simulink model "hw3_a_LMS_model_c0"  (R2024b)
settings: Solver=ode4  StartTime=0.0  StopTime=sim_time  FixedStep=sample_time  RelTol=1e-3
values from neighbouring files (symbols this model uses):
  a = -0.8    [hw3_a_rls_v2.m]    (also in hw3_b_rls_v2.m)
  b = 0.5    [hw3_a_rls_v2.m]    (also in hw3_b_rls_v2.m)
  c = -0.5    [hw3_a_rls_v2.m]    (also in hw3_b_rls_v2.m = 0)
  noise_mean = 0    [hw3_a_rls_v2.m]    (also in hw3_b_rls_v2.m)
  noise_seed = round(rand*1e5)    [hw3_a_rls_v2.m]    (also in hw3_b_rls_v2.m)
  noise_variance = 0.5    [hw3_a_rls_v2.m]    (also in hw3_b_rls_v2.m)
  sample_time = 1    [hw3_a_rls_v2.m]    (also in hw3_b_rls_v2.m)
  Theta_0 = [0;0;0]    [hw3_a_rls_v2.m]    (also in hw3_b_rls_v2.m)
settings Model: Creator=kemal  LastModifiedBy=kemal

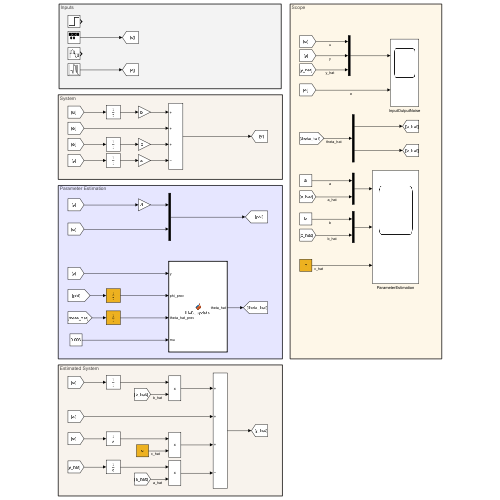
[thumbnail: Simulink's stored preview of the top-level diagram]
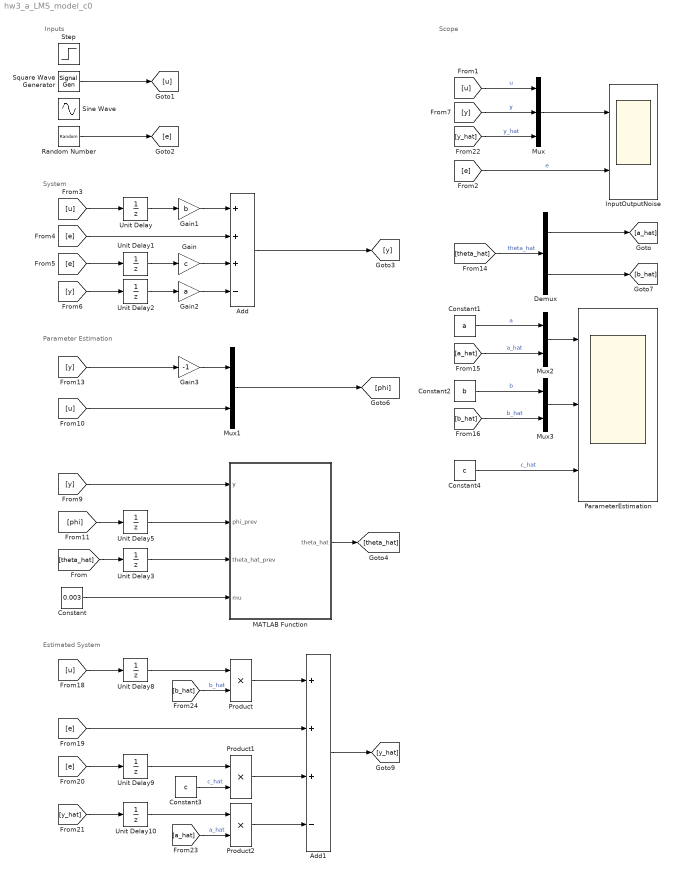
== system hw3_a_LMS_model_c0 ==
  note: Inputs
  note: System
  note: Scope
  note: Parameter Estimation
  note: Estimated System
  Add : Sum  Inputs=+++-
  Add1 : Sum  Inputs=+++-
  Constant : Constant  Value=0.003  SampleTime=sample_time
  Constant1 : Constant  Value=a  SampleTime=sample_time
  Constant2 : Constant  Value=b  SampleTime=sample_time
  Constant3 : Constant  Value=c
  Constant4 : Constant  Value=c
  Demux : Demux  Outputs=2
  Gain : Gain  Gain=c
  Gain1 : Gain  Gain=b
  Gain2 : Gain  Gain=a
  Gain3 : Gain  Gain=-1
  InputOutputNoise : Scope  NumInputPorts=2
  MATLAB Function : MATLAB Function  TreatAsAtomicUnit=on
  Mux : Mux  Inputs=3
  Mux1 : Mux  Inputs=2
  Mux2 : Mux  Inputs=2
  Mux3 : Mux  Inputs=2
  ParameterEstimation : Scope  NumInputPorts=3
  Product : Product
  Product1 : Product
  Product2 : Product
  Random Number : RandomNumber  Mean=noise_mean  Variance=noise_variance  Seed=noise_seed  SampleTime=sample_time
  Sine Wave : Sin  Amplitude=25  Frequency=0.25  SampleTime=sample_time
  Square Wave Generator : SignalGenerator  WaveForm=square  Frequency=1/100
  Step : Step  After=100  SampleTime=0
  Unit Delay{,1..2,5,8..10} (7 alike) : UnitDelay  SampleTime=sample_time  HasFrameUpgradeWarning=on
  Unit Delay3 : UnitDelay  InitialCondition=Theta_0  SampleTime=sample_time  HasFrameUpgradeWarning=on
  wires:
  [u] -> Unit Delay/1
  [e] -> Unit Delay1/1
  Unit Delay1/1 -> Gain/1
  Unit Delay/1 -> Gain1/1
  Gain/1 -> Add/3
  [e] -> Add/2
  Gain1/1 -> Add/1
  [y] -> Unit Delay2/1
  Unit Delay2/1 -> Gain2/1
  Gain2/1 -> Add/4
  Add/1 -> [y]
  Square Wave Generator/1 -> [u]
  [u] -> Mux/1  "u"
  [y] -> Mux/2  "y"
  [e] -> InputOutputNoise/2  "e"
  Mux/1 -> InputOutputNoise/1
  Random Number/1 -> [e]
  MATLAB Function/1(theta_hat) -> [theta_hat]
  [theta_hat] -> Unit Delay3/1
  Unit Delay3/1 -> MATLAB Function/3(theta_hat_prev)
  Constant/1 -> MATLAB Function/4(mu)
  [y] -> MATLAB Function/1(y)
  [y] -> Gain3/1
  Gain3/1 -> Mux1/1
  Mux1/1 -> [phi]
  [phi] -> Unit Delay5/1
  [theta_hat] -> Demux/1  "theta_hat"
  Mux2/1 -> ParameterEstimation/1
  Mux3/1 -> ParameterEstimation/2
  Constant1/1 -> Mux2/1  "a"
  Demux/1 -> [a_hat]
  Demux/2 -> [b_hat]
  Constant2/1 -> Mux3/1  "b"
  [a_hat] -> Mux2/2  "a_hat"
  [b_hat] -> Mux3/2  "b_hat"
  Add1/1 -> [y_hat]
  [y_hat] -> Unit Delay10/1
  Unit Delay8/1 -> Product/1
  [e] -> Unit Delay9/1
  [u] -> Unit Delay8/1
  Product/1 -> Add1/1
  Product1/1 -> Add1/3
  Unit Delay9/1 -> Product1/1
  Product2/1 -> Add1/4
  [b_hat] -> Product/2  "b_hat"
  Constant3/1 -> Product1/2  "c_hat"
  [a_hat] -> Product2/2  "a_hat"
  Unit Delay10/1 -> Product2/1
  [e] -> Add1/2
  [y_hat] -> Mux/3  "y_hat"
  [u] -> Mux1/2
  Unit Delay5/1 -> MATLAB Function/2(phi_prev)
  Constant4/1 -> ParameterEstimation/3  "c_hat"

== matlab function hw3_a_LMS_model_c0/MATLAB Function ==
  data: y input; theta_hat output; phi_prev input; theta_hat_prev input; mu input
function theta_hat  = LMS_update(y, phi_prev, theta_hat_prev, mu)
    % Compute innovation
    epsilon = y - phi_prev' * theta_hat_prev;

    % Update parameter estimate
    theta_hat = theta_hat_prev + mu * phi_prev * epsilon;
end
